simulink model "FinalProject"  (R2021a)
settings: Solver=VariableStepAuto  StartTime=0.0  StopTime=inf  RelTol=1e-3
libraries: vrlib x1
settings Model: Creator=Mulugeta  LastModifiedBy=Mulugeta

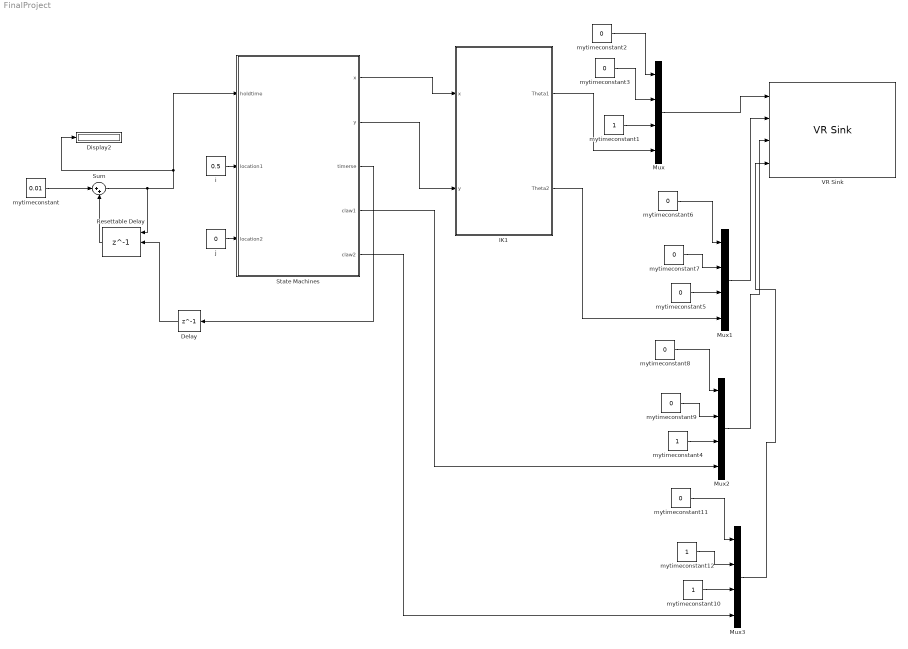
== system FinalProject ==
  Delay : Delay  DelayLength=1  InitialCondition=0
  Display2 : Display
  IK1 : Subsystem
  Mux{,1..3} (4 alike) : Mux
  Resettable Delay : Delay  DelayLength=1  InitialConditionSource=Input port  ExternalReset=Rising
      settings: InputPortMap=u0,r5,p4
  State Machines : Stateflow chart  TreatAsAtomicUnit=on
  Sum : Sum  Inputs=|++
  VR Sink : vrlib/VR Sink  InstantiateOnLoad=on  SampleTime=0.1  ViewEnable=on  RemoteChange=off  RemoteView=off  FieldsWritten=Joint1.rotation.4.1.1.double#joint2.rotation.4.1.1.double#joint4.rotation.4.1.1.double#joint5.rotation.4.1.1.double  WorldFileName=C:\Users\Mulugeta\OneDrive\Desktop\vrealm\FinalProject.WRL  AutoView=off  VideoDimensions=[]  AllowVariableSize=off
  i : Constant  Value=0.5
  j : Constant  Value=0
  mytimeconstant : Constant  Value=0.01
  mytimeconstant{1,4,10,12} (4 alike) : Constant
  mytimeconstant{2..3,5..9,11} (8 alike) : Constant  Value=0
  wires:
  Resettable Delay/1 -> Sum/2
  Sum/1 -> Resettable Delay/1, Display2/1, State Machines/1(holdtime)
  mytimeconstant/1 -> Sum/1
  Delay/1 -> Resettable Delay/2
  State Machines/1(x) -> IK1/1(x)
  State Machines/2(y) -> IK1/2(y)
  i/1 -> State Machines/2(location1)
  j/1 -> State Machines/3(location2)
  mytimeconstant2/1 -> Mux/1
  mytimeconstant3/1 -> Mux/2
  mytimeconstant1/1 -> Mux/3
  IK1/1(Theta1) -> Mux/4
  IK1/2(Theta2) -> Mux1/4
  mytimeconstant5/1 -> Mux1/3
  mytimeconstant7/1 -> Mux1/2
  mytimeconstant6/1 -> Mux1/1
  Mux/1 -> VR Sink/1
  Mux1/1 -> VR Sink/2
  Mux2/1 -> VR Sink/3
  mytimeconstant8/1 -> Mux2/1
  mytimeconstant9/1 -> Mux2/2
  mytimeconstant4/1 -> Mux2/3
  State Machines/3(timerse) -> Delay/1
  State Machines/4(claw1) -> Mux2/4
  State Machines/5(claw2) -> Mux3/4
  mytimeconstant10/1 -> Mux3/3
  mytimeconstant12/1 -> Mux3/2
  mytimeconstant11/1 -> Mux3/1
  Mux3/1 -> VR Sink/4

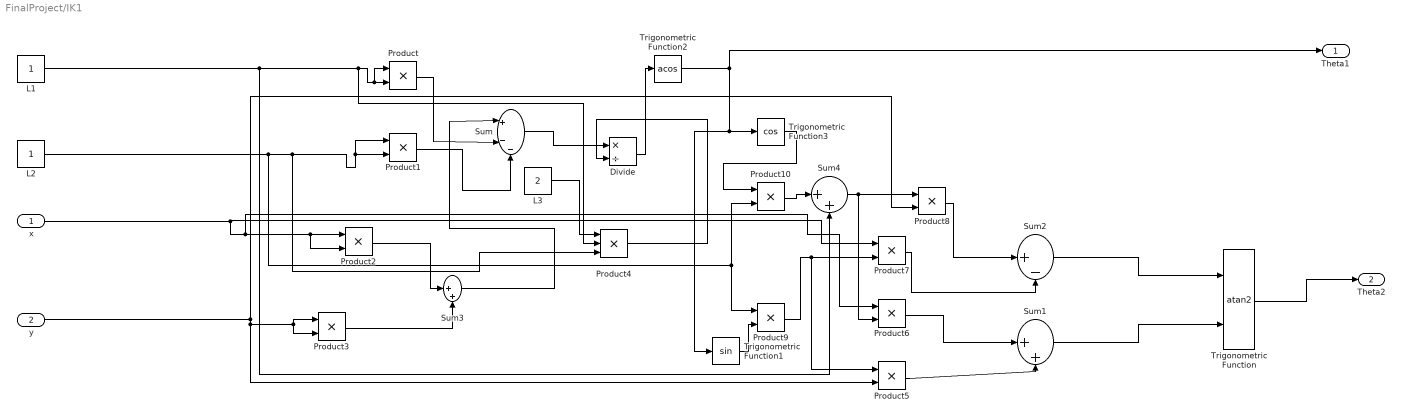
== system FinalProject/IK1 ==
  x : Inport
  y : Inport  Port=2
  Divide : Product  Inputs=*/
  L1 : Constant
  L2 : Constant
  L3 : Constant  Value=2
  Product{,1..3,5..10} (10 alike) : Product
  Product4 : Product  Inputs=3
  Sum : Sum  Inputs=|+--
  Sum1 : Sum  Inputs=|++
  Sum2 : Sum  Inputs=|+-
  Sum3 : Sum  Inputs=|++
  Sum4 : Sum  Inputs=|++
  Trigonometric Function : Trigonometry  Operator=atan2
  Trigonometric Function1 : Trigonometry
  Trigonometric Function2 : Trigonometry  Operator=acos
  Trigonometric Function3 : Trigonometry  Operator=cos
  Theta1 : Outport  VectorParamsAs1DForOutWhenUnconnected=off
  Theta2 : Outport  Port=2  VectorParamsAs1DForOutWhenUnconnected=off
  wires:
  Product9/1 -> Product5/1, Product7/2
  Product5/1 -> Sum1/2
  x/1 -> Product6/1, Product2/2, Product2/1, Product7/1
  Trigonometric Function2/1 -> Theta1/1, Trigonometric Function3/1, Trigonometric Function1/1
  Trigonometric Function1/1 -> Product9/2
  Trigonometric Function3/1 -> Product10/1
  Sum2/1 -> Trigonometric Function/1
  L1/1 -> Sum4/2, Product4/2, Product/1, Product/2
  L2/1 -> Product10/2, Product9/1, Product4/3, Product1/1, Product1/2
  Product4/1 -> Divide/2
  Divide/1 -> Trigonometric Function2/1
  Product10/1 -> Sum4/1
  Sum4/1 -> Product6/2, Product8/1
  Product8/1 -> Sum2/1
  Sum1/1 -> Trigonometric Function/2
  y/1 -> Product5/2, Product3/1, Product3/2, Product8/2
  Product6/1 -> Sum1/1
  Product7/1 -> Sum2/2
  Product1/1 -> Sum/3
  Sum3/1 -> Sum/1
  Product2/1 -> Sum3/1
  Product/1 -> Sum/2
  L3/1 -> Product4/1
  Product3/1 -> Sum3/2
  Sum/1 -> Divide/1
  Trigonometric Function/1 -> Theta2/1

== stateflow chart FinalProject/State Machines ==
  state startstate
    x=0; y=0;timerse=0;claw1=0;claw2=0;
  state holdstate3
    x=0,y=0;timerse=1;
  state centerstate
    x=0,y=0;timerse=0;
  state holdstate2
    x=location1;y=location2;timerse=0;claw1=3.14/2; claw2=3.14/2;
  state holdstate1
    x=0;y=0;timerse=0;
  state graspstate
    x=location1;y=location2;timerse=0;claw1=3.14/2; claw2=3.14/2;
  state targetpostion
    x=location1,y=location2;timerse=0;
  state holdstate4
    x=location1;y=location2;timerse=0;
  (default) -> startstate
  holdstate3 -> centerstate
  startstate -> centerstate
  holdstate2 -> holdstate3 : [x<=0 && y<=0]
  centerstate -> holdstate1 : [holdtime > 25]
  graspstate -> holdstate2 : [holdtime > 150]
  holdstate1 -> targetpostion : [x >=location1 &&y >= location2]
  holdstate4 -> graspstate
  targetpostion -> holdstate4 : [holdtime > 75]
  data: x output; y output; holdtime input; timerse output; location1 input; location2 input; claw1 output; claw2 output
